simulink model "NeuronalNetwork"  (R2019b)
(part 11 of 11)

  dotprod426/1 -> Mux/426
  "IW{2,1}(427,:)'"/1 -> dotprod427/1
  dotprod427/1 -> Mux/427
  "IW{2,1}(428,:)'"/1 -> dotprod428/1
  dotprod428/1 -> Mux/428
  "IW{2,1}(429,:)'"/1 -> dotprod429/1
  dotprod429/1 -> Mux/429
  "IW{2,1}(430,:)'"/1 -> dotprod430/1
  dotprod430/1 -> Mux/430
  "IW{2,1}(431,:)'"/1 -> dotprod431/1
  dotprod431/1 -> Mux/431
  "IW{2,1}(432,:)'"/1 -> dotprod432/1
  dotprod432/1 -> Mux/432
  "IW{2,1}(433,:)'"/1 -> dotprod433/1
  dotprod433/1 -> Mux/433
  "IW{2,1}(434,:)'"/1 -> dotprod434/1
  dotprod434/1 -> Mux/434
  "IW{2,1}(435,:)'"/1 -> dotprod435/1
  dotprod435/1 -> Mux/435
  "IW{2,1}(436,:)'"/1 -> dotprod436/1
  dotprod436/1 -> Mux/436
  "IW{2,1}(437,:)'"/1 -> dotprod437/1
  dotprod437/1 -> Mux/437
  "IW{2,1}(438,:)'"/1 -> dotprod438/1
  dotprod438/1 -> Mux/438
  "IW{2,1}(439,:)'"/1 -> dotprod439/1
  dotprod439/1 -> Mux/439
  "IW{2,1}(440,:)'"/1 -> dotprod440/1
  dotprod440/1 -> Mux/440
  "IW{2,1}(441,:)'"/1 -> dotprod441/1
  dotprod441/1 -> Mux/441
  "IW{2,1}(442,:)'"/1 -> dotprod442/1
  dotprod442/1 -> Mux/442
  "IW{2,1}(443,:)'"/1 -> dotprod443/1
  dotprod443/1 -> Mux/443
  "IW{2,1}(444,:)'"/1 -> dotprod444/1
  dotprod444/1 -> Mux/444
  "IW{2,1}(445,:)'"/1 -> dotprod445/1
  dotprod445/1 -> Mux/445
  "IW{2,1}(446,:)'"/1 -> dotprod446/1
  dotprod446/1 -> Mux/446
  "IW{2,1}(447,:)'"/1 -> dotprod447/1
  dotprod447/1 -> Mux/447
  "IW{2,1}(448,:)'"/1 -> dotprod448/1
  dotprod448/1 -> Mux/448
  "IW{2,1}(449,:)'"/1 -> dotprod449/1
  dotprod449/1 -> Mux/449
  "IW{2,1}(450,:)'"/1 -> dotprod450/1
  dotprod450/1 -> Mux/450
  "IW{2,1}(451,:)'"/1 -> dotprod451/1
  dotprod451/1 -> Mux/451
  "IW{2,1}(452,:)'"/1 -> dotprod452/1
  dotprod452/1 -> Mux/452
  "IW{2,1}(453,:)'"/1 -> dotprod453/1
  dotprod453/1 -> Mux/453
  "IW{2,1}(454,:)'"/1 -> dotprod454/1
  dotprod454/1 -> Mux/454
  "IW{2,1}(455,:)'"/1 -> dotprod455/1
  dotprod455/1 -> Mux/455
  "IW{2,1}(456,:)'"/1 -> dotprod456/1
  dotprod456/1 -> Mux/456
  "IW{2,1}(457,:)'"/1 -> dotprod457/1
  dotprod457/1 -> Mux/457
  "IW{2,1}(458,:)'"/1 -> dotprod458/1
  dotprod458/1 -> Mux/458
  "IW{2,1}(459,:)'"/1 -> dotprod459/1
  dotprod459/1 -> Mux/459
  "IW{2,1}(460,:)'"/1 -> dotprod460/1
  dotprod460/1 -> Mux/460
  "IW{2,1}(461,:)'"/1 -> dotprod461/1
  dotprod461/1 -> Mux/461
  "IW{2,1}(462,:)'"/1 -> dotprod462/1
  dotprod462/1 -> Mux/462
  "IW{2,1}(463,:)'"/1 -> dotprod463/1
  dotprod463/1 -> Mux/463
  "IW{2,1}(464,:)'"/1 -> dotprod464/1
  dotprod464/1 -> Mux/464
  "IW{2,1}(465,:)'"/1 -> dotprod465/1
  dotprod465/1 -> Mux/465
  "IW{2,1}(466,:)'"/1 -> dotprod466/1
  dotprod466/1 -> Mux/466
  "IW{2,1}(467,:)'"/1 -> dotprod467/1
  dotprod467/1 -> Mux/467
  "IW{2,1}(468,:)'"/1 -> dotprod468/1
  dotprod468/1 -> Mux/468
  "IW{2,1}(469,:)'"/1 -> dotprod469/1
  dotprod469/1 -> Mux/469
  "IW{2,1}(470,:)'"/1 -> dotprod470/1
  dotprod470/1 -> Mux/470
  "IW{2,1}(471,:)'"/1 -> dotprod471/1
  dotprod471/1 -> Mux/471
  "IW{2,1}(472,:)'"/1 -> dotprod472/1
  dotprod472/1 -> Mux/472
  "IW{2,1}(473,:)'"/1 -> dotprod473/1
  dotprod473/1 -> Mux/473
  "IW{2,1}(474,:)'"/1 -> dotprod474/1
  dotprod474/1 -> Mux/474
  "IW{2,1}(475,:)'"/1 -> dotprod475/1
  dotprod475/1 -> Mux/475
  "IW{2,1}(476,:)'"/1 -> dotprod476/1
  dotprod476/1 -> Mux/476
  "IW{2,1}(477,:)'"/1 -> dotprod477/1
  dotprod477/1 -> Mux/477
  "IW{2,1}(478,:)'"/1 -> dotprod478/1
  dotprod478/1 -> Mux/478
  "IW{2,1}(479,:)'"/1 -> dotprod479/1
  dotprod479/1 -> Mux/479
  "IW{2,1}(480,:)'"/1 -> dotprod480/1
  dotprod480/1 -> Mux/480
  "IW{2,1}(481,:)'"/1 -> dotprod481/1
  dotprod481/1 -> Mux/481
  "IW{2,1}(482,:)'"/1 -> dotprod482/1
  dotprod482/1 -> Mux/482
  "IW{2,1}(483,:)'"/1 -> dotprod483/1
  dotprod483/1 -> Mux/483
  "IW{2,1}(484,:)'"/1 -> dotprod484/1
  dotprod484/1 -> Mux/484
  "IW{2,1}(485,:)'"/1 -> dotprod485/1
  dotprod485/1 -> Mux/485
  "IW{2,1}(486,:)'"/1 -> dotprod486/1
  dotprod486/1 -> Mux/486
  "IW{2,1}(487,:)'"/1 -> dotprod487/1
  dotprod487/1 -> Mux/487
  "IW{2,1}(488,:)'"/1 -> dotprod488/1
  dotprod488/1 -> Mux/488
  "IW{2,1}(489,:)'"/1 -> dotprod489/1
  dotprod489/1 -> Mux/489
  "IW{2,1}(490,:)'"/1 -> dotprod490/1
  dotprod490/1 -> Mux/490
  "IW{2,1}(491,:)'"/1 -> dotprod491/1
  dotprod491/1 -> Mux/491
  "IW{2,1}(492,:)'"/1 -> dotprod492/1
  dotprod492/1 -> Mux/492
  "IW{2,1}(493,:)'"/1 -> dotprod493/1
  dotprod493/1 -> Mux/493
  "IW{2,1}(494,:)'"/1 -> dotprod494/1
  dotprod494/1 -> Mux/494
  "IW{2,1}(495,:)'"/1 -> dotprod495/1
  dotprod495/1 -> Mux/495
  "IW{2,1}(496,:)'"/1 -> dotprod496/1
  dotprod496/1 -> Mux/496
  "IW{2,1}(497,:)'"/1 -> dotprod497/1
  dotprod497/1 -> Mux/497
  "IW{2,1}(498,:)'"/1 -> dotprod498/1
  dotprod498/1 -> Mux/498
  "IW{2,1}(499,:)'"/1 -> dotprod499/1
  dotprod499/1 -> Mux/499
  "IW{2,1}(500,:)'"/1 -> dotprod500/1
  dotprod500/1 -> Mux/500
  "IW{2,1}(501,:)'"/1 -> dotprod501/1
  dotprod501/1 -> Mux/501
  "IW{2,1}(502,:)'"/1 -> dotprod502/1
  dotprod502/1 -> Mux/502
  "IW{2,1}(503,:)'"/1 -> dotprod503/1
  dotprod503/1 -> Mux/503
  "IW{2,1}(504,:)'"/1 -> dotprod504/1
  dotprod504/1 -> Mux/504
  "IW{2,1}(505,:)'"/1 -> dotprod505/1
  dotprod505/1 -> Mux/505
  "IW{2,1}(506,:)'"/1 -> dotprod506/1
  dotprod506/1 -> Mux/506
  "IW{2,1}(507,:)'"/1 -> dotprod507/1
  dotprod507/1 -> Mux/507
  "IW{2,1}(508,:)'"/1 -> dotprod508/1
  dotprod508/1 -> Mux/508
  "IW{2,1}(509,:)'"/1 -> dotprod509/1
  dotprod509/1 -> Mux/509
  "IW{2,1}(510,:)'"/1 -> dotprod510/1
  dotprod510/1 -> Mux/510
  "IW{2,1}(511,:)'"/1 -> dotprod511/1
  dotprod511/1 -> Mux/511
  "IW{2,1}(512,:)'"/1 -> dotprod512/1
  dotprod512/1 -> Mux/512
  "IW{2,1}(513,:)'"/1 -> dotprod513/1
  dotprod513/1 -> Mux/513
  "IW{2,1}(514,:)'"/1 -> dotprod514/1
  dotprod514/1 -> Mux/514
  "IW{2,1}(515,:)'"/1 -> dotprod515/1
  dotprod515/1 -> Mux/515
  "IW{2,1}(516,:)'"/1 -> dotprod516/1
  dotprod516/1 -> Mux/516
  "IW{2,1}(517,:)'"/1 -> dotprod517/1
  dotprod517/1 -> Mux/517
  "IW{2,1}(518,:)'"/1 -> dotprod518/1
  dotprod518/1 -> Mux/518
  "IW{2,1}(519,:)'"/1 -> dotprod519/1
  dotprod519/1 -> Mux/519
  "IW{2,1}(520,:)'"/1 -> dotprod520/1
  dotprod520/1 -> Mux/520
  "IW{2,1}(521,:)'"/1 -> dotprod521/1
  dotprod521/1 -> Mux/521
  "IW{2,1}(522,:)'"/1 -> dotprod522/1
  dotprod522/1 -> Mux/522
  "IW{2,1}(523,:)'"/1 -> dotprod523/1
  dotprod523/1 -> Mux/523
  "IW{2,1}(524,:)'"/1 -> dotprod524/1
  dotprod524/1 -> Mux/524
  "IW{2,1}(525,:)'"/1 -> dotprod525/1
  dotprod525/1 -> Mux/525
  "IW{2,1}(526,:)'"/1 -> dotprod526/1
  dotprod526/1 -> Mux/526
  "IW{2,1}(527,:)'"/1 -> dotprod527/1
  dotprod527/1 -> Mux/527
  "IW{2,1}(528,:)'"/1 -> dotprod528/1
  dotprod528/1 -> Mux/528
  "IW{2,1}(529,:)'"/1 -> dotprod529/1
  dotprod529/1 -> Mux/529
  "IW{2,1}(530,:)'"/1 -> dotprod530/1
  dotprod530/1 -> Mux/530
  "IW{2,1}(531,:)'"/1 -> dotprod531/1
  dotprod531/1 -> Mux/531
  "IW{2,1}(532,:)'"/1 -> dotprod532/1
  dotprod532/1 -> Mux/532
  "IW{2,1}(533,:)'"/1 -> dotprod533/1
  dotprod533/1 -> Mux/533
  "IW{2,1}(534,:)'"/1 -> dotprod534/1
  dotprod534/1 -> Mux/534
  "IW{2,1}(535,:)'"/1 -> dotprod535/1
  dotprod535/1 -> Mux/535
  "IW{2,1}(536,:)'"/1 -> dotprod536/1
  dotprod536/1 -> Mux/536
  "IW{2,1}(537,:)'"/1 -> dotprod537/1
  dotprod537/1 -> Mux/537
  "IW{2,1}(538,:)'"/1 -> dotprod538/1
  dotprod538/1 -> Mux/538
  "IW{2,1}(539,:)'"/1 -> dotprod539/1
  dotprod539/1 -> Mux/539
  "IW{2,1}(540,:)'"/1 -> dotprod540/1
  dotprod540/1 -> Mux/540
  "IW{2,1}(541,:)'"/1 -> dotprod541/1
  dotprod541/1 -> Mux/541
  "IW{2,1}(542,:)'"/1 -> dotprod542/1
  dotprod542/1 -> Mux/542
  "IW{2,1}(543,:)'"/1 -> dotprod543/1
  dotprod543/1 -> Mux/543
  "IW{2,1}(544,:)'"/1 -> dotprod544/1
  dotprod544/1 -> Mux/544
  "IW{2,1}(545,:)'"/1 -> dotprod545/1
  dotprod545/1 -> Mux/545
  "IW{2,1}(546,:)'"/1 -> dotprod546/1
  dotprod546/1 -> Mux/546
  "IW{2,1}(547,:)'"/1 -> dotprod547/1
  dotprod547/1 -> Mux/547
  "IW{2,1}(548,:)'"/1 -> dotprod548/1
  dotprod548/1 -> Mux/548
  "IW{2,1}(549,:)'"/1 -> dotprod549/1
  dotprod549/1 -> Mux/549
  "IW{2,1}(550,:)'"/1 -> dotprod550/1
  dotprod550/1 -> Mux/550
  "IW{2,1}(551,:)'"/1 -> dotprod551/1
  dotprod551/1 -> Mux/551
  "IW{2,1}(552,:)'"/1 -> dotprod552/1
  dotprod552/1 -> Mux/552
  "IW{2,1}(553,:)'"/1 -> dotprod553/1
  dotprod553/1 -> Mux/553
  "IW{2,1}(554,:)'"/1 -> dotprod554/1
  dotprod554/1 -> Mux/554
  "IW{2,1}(555,:)'"/1 -> dotprod555/1
  dotprod555/1 -> Mux/555
  "IW{2,1}(556,:)'"/1 -> dotprod556/1
  dotprod556/1 -> Mux/556
  "IW{2,1}(557,:)'"/1 -> dotprod557/1
  dotprod557/1 -> Mux/557
  "IW{2,1}(558,:)'"/1 -> dotprod558/1
  dotprod558/1 -> Mux/558
  "IW{2,1}(559,:)'"/1 -> dotprod559/1
  dotprod559/1 -> Mux/559
  "IW{2,1}(560,:)'"/1 -> dotprod560/1
  dotprod560/1 -> Mux/560
  "IW{2,1}(561,:)'"/1 -> dotprod561/1
  dotprod561/1 -> Mux/561
  "IW{2,1}(562,:)'"/1 -> dotprod562/1
  dotprod562/1 -> Mux/562
  "IW{2,1}(563,:)'"/1 -> dotprod563/1
  dotprod563/1 -> Mux/563
  "IW{2,1}(564,:)'"/1 -> dotprod564/1
  dotprod564/1 -> Mux/564
  "IW{2,1}(565,:)'"/1 -> dotprod565/1
  dotprod565/1 -> Mux/565
  "IW{2,1}(566,:)'"/1 -> dotprod566/1
  dotprod566/1 -> Mux/566
  "IW{2,1}(567,:)'"/1 -> dotprod567/1
  dotprod567/1 -> Mux/567
  "IW{2,1}(568,:)'"/1 -> dotprod568/1
  dotprod568/1 -> Mux/568
  "IW{2,1}(569,:)'"/1 -> dotprod569/1
  dotprod569/1 -> Mux/569
  "IW{2,1}(570,:)'"/1 -> dotprod570/1
  dotprod570/1 -> Mux/570
  "IW{2,1}(571,:)'"/1 -> dotprod571/1
  dotprod571/1 -> Mux/571
  "IW{2,1}(572,:)'"/1 -> dotprod572/1
  dotprod572/1 -> Mux/572
  "IW{2,1}(573,:)'"/1 -> dotprod573/1
  dotprod573/1 -> Mux/573
  "IW{2,1}(574,:)'"/1 -> dotprod574/1
  dotprod574/1 -> Mux/574
  "IW{2,1}(575,:)'"/1 -> dotprod575/1
  dotprod575/1 -> Mux/575
  "IW{2,1}(576,:)'"/1 -> dotprod576/1
  dotprod576/1 -> Mux/576
  "IW{2,1}(577,:)'"/1 -> dotprod577/1
  dotprod577/1 -> Mux/577
  "IW{2,1}(578,:)'"/1 -> dotprod578/1
  dotprod578/1 -> Mux/578
  "IW{2,1}(579,:)'"/1 -> dotprod579/1
  dotprod579/1 -> Mux/579
  "IW{2,1}(580,:)'"/1 -> dotprod580/1
  dotprod580/1 -> Mux/580
  "IW{2,1}(581,:)'"/1 -> dotprod581/1
  dotprod581/1 -> Mux/581
  "IW{2,1}(582,:)'"/1 -> dotprod582/1
  dotprod582/1 -> Mux/582
  "IW{2,1}(583,:)'"/1 -> dotprod583/1
  dotprod583/1 -> Mux/583
  "IW{2,1}(584,:)'"/1 -> dotprod584/1
  dotprod584/1 -> Mux/584
  "IW{2,1}(585,:)'"/1 -> dotprod585/1
  dotprod585/1 -> Mux/585
  "IW{2,1}(586,:)'"/1 -> dotprod586/1
  dotprod586/1 -> Mux/586
  "IW{2,1}(587,:)'"/1 -> dotprod587/1
  dotprod587/1 -> Mux/587
  "IW{2,1}(588,:)'"/1 -> dotprod588/1
  dotprod588/1 -> Mux/588
  "IW{2,1}(589,:)'"/1 -> dotprod589/1
  dotprod589/1 -> Mux/589
  "IW{2,1}(590,:)'"/1 -> dotprod590/1
  dotprod590/1 -> Mux/590
  "IW{2,1}(591,:)'"/1 -> dotprod591/1
  dotprod591/1 -> Mux/591
  "IW{2,1}(592,:)'"/1 -> dotprod592/1
  dotprod592/1 -> Mux/592
  "IW{2,1}(593,:)'"/1 -> dotprod593/1
  dotprod593/1 -> Mux/593
  "IW{2,1}(594,:)'"/1 -> dotprod594/1
  dotprod594/1 -> Mux/594
  "IW{2,1}(595,:)'"/1 -> dotprod595/1
  dotprod595/1 -> Mux/595
  "IW{2,1}(596,:)'"/1 -> dotprod596/1
  dotprod596/1 -> Mux/596
  "IW{2,1}(597,:)'"/1 -> dotprod597/1
  dotprod597/1 -> Mux/597
  "IW{2,1}(598,:)'"/1 -> dotprod598/1
  dotprod598/1 -> Mux/598
  "IW{2,1}(599,:)'"/1 -> dotprod599/1
  dotprod599/1 -> Mux/599
  "IW{2,1}(600,:)'"/1 -> dotprod600/1
  dotprod600/1 -> Mux/600
  "IW{2,1}(601,:)'"/1 -> dotprod601/1
  dotprod601/1 -> Mux/601
  "IW{2,1}(602,:)'"/1 -> dotprod602/1
  dotprod602/1 -> Mux/602
  "IW{2,1}(603,:)'"/1 -> dotprod603/1
  dotprod603/1 -> Mux/603
  "IW{2,1}(604,:)'"/1 -> dotprod604/1
  dotprod604/1 -> Mux/604
  "IW{2,1}(605,:)'"/1 -> dotprod605/1
  dotprod605/1 -> Mux/605
  "IW{2,1}(606,:)'"/1 -> dotprod606/1
  dotprod606/1 -> Mux/606
  "IW{2,1}(607,:)'"/1 -> dotprod607/1
  dotprod607/1 -> Mux/607
  "IW{2,1}(608,:)'"/1 -> dotprod608/1
  dotprod608/1 -> Mux/608
  "IW{2,1}(609,:)'"/1 -> dotprod609/1
  dotprod609/1 -> Mux/609
  "IW{2,1}(610,:)'"/1 -> dotprod610/1
  dotprod610/1 -> Mux/610
  "IW{2,1}(611,:)'"/1 -> dotprod611/1
  dotprod611/1 -> Mux/611
  "IW{2,1}(612,:)'"/1 -> dotprod612/1
  dotprod612/1 -> Mux/612
  "IW{2,1}(613,:)'"/1 -> dotprod613/1
  dotprod613/1 -> Mux/613
  "IW{2,1}(614,:)'"/1 -> dotprod614/1
  dotprod614/1 -> Mux/614
  "IW{2,1}(615,:)'"/1 -> dotprod615/1
  dotprod615/1 -> Mux/615
  "IW{2,1}(616,:)'"/1 -> dotprod616/1
  dotprod616/1 -> Mux/616
  "IW{2,1}(617,:)'"/1 -> dotprod617/1
  dotprod617/1 -> Mux/617
  "IW{2,1}(618,:)'"/1 -> dotprod618/1
  dotprod618/1 -> Mux/618
  "IW{2,1}(619,:)'"/1 -> dotprod619/1
  dotprod619/1 -> Mux/619
  "IW{2,1}(620,:)'"/1 -> dotprod620/1
  dotprod620/1 -> Mux/620
  "IW{2,1}(621,:)'"/1 -> dotprod621/1
  dotprod621/1 -> Mux/621
  "IW{2,1}(622,:)'"/1 -> dotprod622/1
  dotprod622/1 -> Mux/622
  "IW{2,1}(623,:)'"/1 -> dotprod623/1
  dotprod623/1 -> Mux/623
  "IW{2,1}(624,:)'"/1 -> dotprod624/1
  dotprod624/1 -> Mux/624
  "IW{2,1}(625,:)'"/1 -> dotprod625/1
  dotprod625/1 -> Mux/625
  "IW{2,1}(626,:)'"/1 -> dotprod626/1
  dotprod626/1 -> Mux/626
  "IW{2,1}(627,:)'"/1 -> dotprod627/1
  dotprod627/1 -> Mux/627
  "IW{2,1}(628,:)'"/1 -> dotprod628/1
  dotprod628/1 -> Mux/628
  "IW{2,1}(629,:)'"/1 -> dotprod629/1
  dotprod629/1 -> Mux/629
  "IW{2,1}(630,:)'"/1 -> dotprod630/1
  dotprod630/1 -> Mux/630
  "IW{2,1}(631,:)'"/1 -> dotprod631/1
  dotprod631/1 -> Mux/631
  "IW{2,1}(632,:)'"/1 -> dotprod632/1
  dotprod632/1 -> Mux/632
  "IW{2,1}(633,:)'"/1 -> dotprod633/1
  dotprod633/1 -> Mux/633
  "IW{2,1}(634,:)'"/1 -> dotprod634/1
  dotprod634/1 -> Mux/634
  "IW{2,1}(635,:)'"/1 -> dotprod635/1
  dotprod635/1 -> Mux/635
  "IW{2,1}(636,:)'"/1 -> dotprod636/1
  dotprod636/1 -> Mux/636
  "IW{2,1}(637,:)'"/1 -> dotprod637/1
  dotprod637/1 -> Mux/637
  "IW{2,1}(638,:)'"/1 -> dotprod638/1
  dotprod638/1 -> Mux/638
  "IW{2,1}(639,:)'"/1 -> dotprod639/1
  dotprod639/1 -> Mux/639
  "IW{2,1}(640,:)'"/1 -> dotprod640/1
  dotprod640/1 -> Mux/640
  "IW{2,1}(641,:)'"/1 -> dotprod641/1
  dotprod641/1 -> Mux/641
  "IW{2,1}(642,:)'"/1 -> dotprod642/1
  dotprod642/1 -> Mux/642
  "IW{2,1}(643,:)'"/1 -> dotprod643/1
  dotprod643/1 -> Mux/643
  "IW{2,1}(644,:)'"/1 -> dotprod644/1
  dotprod644/1 -> Mux/644
  "IW{2,1}(645,:)'"/1 -> dotprod645/1
  dotprod645/1 -> Mux/645
  "IW{2,1}(646,:)'"/1 -> dotprod646/1
  dotprod646/1 -> Mux/646
  "IW{2,1}(647,:)'"/1 -> dotprod647/1
  dotprod647/1 -> Mux/647
  "IW{2,1}(648,:)'"/1 -> dotprod648/1
  dotprod648/1 -> Mux/648
  "IW{2,1}(649,:)'"/1 -> dotprod649/1
  dotprod649/1 -> Mux/649
  "IW{2,1}(650,:)'"/1 -> dotprod650/1
  dotprod650/1 -> Mux/650
  "IW{2,1}(651,:)'"/1 -> dotprod651/1
  dotprod651/1 -> Mux/651
  "IW{2,1}(652,:)'"/1 -> dotprod652/1
  dotprod652/1 -> Mux/652
  "IW{2,1}(653,:)'"/1 -> dotprod653/1
  dotprod653/1 -> Mux/653
  "IW{2,1}(654,:)'"/1 -> dotprod654/1
  dotprod654/1 -> Mux/654
  "IW{2,1}(655,:)'"/1 -> dotprod655/1
  dotprod655/1 -> Mux/655
  "IW{2,1}(656,:)'"/1 -> dotprod656/1
  dotprod656/1 -> Mux/656
  "IW{2,1}(657,:)'"/1 -> dotprod657/1
  dotprod657/1 -> Mux/657
  "IW{2,1}(658,:)'"/1 -> dotprod658/1
  dotprod658/1 -> Mux/658
  "IW{2,1}(659,:)'"/1 -> dotprod659/1
  dotprod659/1 -> Mux/659
  "IW{2,1}(660,:)'"/1 -> dotprod660/1
  dotprod660/1 -> Mux/660
  "IW{2,1}(661,:)'"/1 -> dotprod661/1
  dotprod661/1 -> Mux/661
  "IW{2,1}(662,:)'"/1 -> dotprod662/1
  dotprod662/1 -> Mux/662
  "IW{2,1}(663,:)'"/1 -> dotprod663/1
  dotprod663/1 -> Mux/663
  "IW{2,1}(664,:)'"/1 -> dotprod664/1
  dotprod664/1 -> Mux/664
  "IW{2,1}(665,:)'"/1 -> dotprod665/1
  dotprod665/1 -> Mux/665
  "IW{2,1}(666,:)'"/1 -> dotprod666/1
  dotprod666/1 -> Mux/666
  "IW{2,1}(667,:)'"/1 -> dotprod667/1
  dotprod667/1 -> Mux/667
  "IW{2,1}(668,:)'"/1 -> dotprod668/1
  dotprod668/1 -> Mux/668
  "IW{2,1}(669,:)'"/1 -> dotprod669/1
  dotprod669/1 -> Mux/669
  "IW{2,1}(670,:)'"/1 -> dotprod670/1
  dotprod670/1 -> Mux/670
  "IW{2,1}(671,:)'"/1 -> dotprod671/1
  dotprod671/1 -> Mux/671
  "IW{2,1}(672,:)'"/1 -> dotprod672/1
  dotprod672/1 -> Mux/672
  "IW{2,1}(673,:)'"/1 -> dotprod673/1
  dotprod673/1 -> Mux/673
  "IW{2,1}(674,:)'"/1 -> dotprod674/1
  dotprod674/1 -> Mux/674
  "IW{2,1}(675,:)'"/1 -> dotprod675/1
  dotprod675/1 -> Mux/675
  "IW{2,1}(676,:)'"/1 -> dotprod676/1
  dotprod676/1 -> Mux/676
  "IW{2,1}(677,:)'"/1 -> dotprod677/1
  dotprod677/1 -> Mux/677
  "IW{2,1}(678,:)'"/1 -> dotprod678/1
  dotprod678/1 -> Mux/678
  "IW{2,1}(679,:)'"/1 -> dotprod679/1
  dotprod679/1 -> Mux/679
  "IW{2,1}(680,:)'"/1 -> dotprod680/1
  dotprod680/1 -> Mux/680
  "IW{2,1}(681,:)'"/1 -> dotprod681/1
  dotprod681/1 -> Mux/681
  "IW{2,1}(682,:)'"/1 -> dotprod682/1
  dotprod682/1 -> Mux/682
  "IW{2,1}(683,:)'"/1 -> dotprod683/1
  dotprod683/1 -> Mux/683
  "IW{2,1}(684,:)'"/1 -> dotprod684/1
  dotprod684/1 -> Mux/684
  "IW{2,1}(685,:)'"/1 -> dotprod685/1
  dotprod685/1 -> Mux/685
  "IW{2,1}(686,:)'"/1 -> dotprod686/1
  dotprod686/1 -> Mux/686
  "IW{2,1}(687,:)'"/1 -> dotprod687/1
  dotprod687/1 -> Mux/687
  "IW{2,1}(688,:)'"/1 -> dotprod688/1
  dotprod688/1 -> Mux/688
  "IW{2,1}(689,:)'"/1 -> dotprod689/1
  dotprod689/1 -> Mux/689
  "IW{2,1}(690,:)'"/1 -> dotprod690/1
  dotprod690/1 -> Mux/690
  "IW{2,1}(691,:)'"/1 -> dotprod691/1
  dotprod691/1 -> Mux/691
  "IW{2,1}(692,:)'"/1 -> dotprod692/1
  dotprod692/1 -> Mux/692
  "IW{2,1}(693,:)'"/1 -> dotprod693/1
  dotprod693/1 -> Mux/693
  "IW{2,1}(694,:)'"/1 -> dotprod694/1
  dotprod694/1 -> Mux/694
  "IW{2,1}(695,:)'"/1 -> dotprod695/1
  dotprod695/1 -> Mux/695
  "IW{2,1}(696,:)'"/1 -> dotprod696/1
  dotprod696/1 -> Mux/696
  "IW{2,1}(697,:)'"/1 -> dotprod697/1
  dotprod697/1 -> Mux/697
  "IW{2,1}(698,:)'"/1 -> dotprod698/1
  dotprod698/1 -> Mux/698
  "IW{2,1}(699,:)'"/1 -> dotprod699/1
  dotprod699/1 -> Mux/699
  "IW{2,1}(700,:)'"/1 -> dotprod700/1
  dotprod700/1 -> Mux/700
  "IW{2,1}(701,:)'"/1 -> dotprod701/1
  dotprod701/1 -> Mux/701
  "IW{2,1}(702,:)'"/1 -> dotprod702/1
  dotprod702/1 -> Mux/702
  "IW{2,1}(703,:)'"/1 -> dotprod703/1
  dotprod703/1 -> Mux/703
  "IW{2,1}(704,:)'"/1 -> dotprod704/1
  dotprod704/1 -> Mux/704
  "IW{2,1}(705,:)'"/1 -> dotprod705/1
  dotprod705/1 -> Mux/705
  "IW{2,1}(706,:)'"/1 -> dotprod706/1
  dotprod706/1 -> Mux/706
  "IW{2,1}(707,:)'"/1 -> dotprod707/1
  dotprod707/1 -> Mux/707
  "IW{2,1}(708,:)'"/1 -> dotprod708/1
  dotprod708/1 -> Mux/708
  "IW{2,1}(709,:)'"/1 -> dotprod709/1
  dotprod709/1 -> Mux/709
  "IW{2,1}(710,:)'"/1 -> dotprod710/1
  dotprod710/1 -> Mux/710
  "IW{2,1}(711,:)'"/1 -> dotprod711/1
  dotprod711/1 -> Mux/711
  "IW{2,1}(712,:)'"/1 -> dotprod712/1
  dotprod712/1 -> Mux/712
  "IW{2,1}(713,:)'"/1 -> dotprod713/1
  dotprod713/1 -> Mux/713
  "IW{2,1}(714,:)'"/1 -> dotprod714/1
  dotprod714/1 -> Mux/714
  "IW{2,1}(715,:)'"/1 -> dotprod715/1
  dotprod715/1 -> Mux/715
  "IW{2,1}(716,:)'"/1 -> dotprod716/1
  dotprod716/1 -> Mux/716
  "IW{2,1}(717,:)'"/1 -> dotprod717/1
  dotprod717/1 -> Mux/717
  "IW{2,1}(718,:)'"/1 -> dotprod718/1
  dotprod718/1 -> Mux/718
  "IW{2,1}(719,:)'"/1 -> dotprod719/1
  dotprod719/1 -> Mux/719
  "IW{2,1}(720,:)'"/1 -> dotprod720/1
  dotprod720/1 -> Mux/720
  "IW{2,1}(721,:)'"/1 -> dotprod721/1
  dotprod721/1 -> Mux/721
  "IW{2,1}(722,:)'"/1 -> dotprod722/1
  dotprod722/1 -> Mux/722
  "IW{2,1}(723,:)'"/1 -> dotprod723/1
  dotprod723/1 -> Mux/723
  "IW{2,1}(724,:)'"/1 -> dotprod724/1
  dotprod724/1 -> Mux/724
  "IW{2,1}(725,:)'"/1 -> dotprod725/1
  dotprod725/1 -> Mux/725
  "IW{2,1}(726,:)'"/1 -> dotprod726/1
  dotprod726/1 -> Mux/726
  "IW{2,1}(727,:)'"/1 -> dotprod727/1
  dotprod727/1 -> Mux/727
  "IW{2,1}(728,:)'"/1 -> dotprod728/1
  dotprod728/1 -> Mux/728
  "IW{2,1}(729,:)'"/1 -> dotprod729/1
  dotprod729/1 -> Mux/729
  "IW{2,1}(730,:)'"/1 -> dotprod730/1
  dotprod730/1 -> Mux/730
  "IW{2,1}(731,:)'"/1 -> dotprod731/1
  dotprod731/1 -> Mux/731
  "IW{2,1}(732,:)'"/1 -> dotprod732/1
  dotprod732/1 -> Mux/732
  "IW{2,1}(733,:)'"/1 -> dotprod733/1
  dotprod733/1 -> Mux/733
  "IW{2,1}(734,:)'"/1 -> dotprod734/1
  dotprod734/1 -> Mux/734
  "IW{2,1}(735,:)'"/1 -> dotprod735/1
  dotprod735/1 -> Mux/735
  "IW{2,1}(736,:)'"/1 -> dotprod736/1
  dotprod736/1 -> Mux/736
  "IW{2,1}(737,:)'"/1 -> dotprod737/1
  dotprod737/1 -> Mux/737
  "IW{2,1}(738,:)'"/1 -> dotprod738/1
  dotprod738/1 -> Mux/738
  "IW{2,1}(739,:)'"/1 -> dotprod739/1
  dotprod739/1 -> Mux/739
  "IW{2,1}(740,:)'"/1 -> dotprod740/1
  dotprod740/1 -> Mux/740
  "IW{2,1}(741,:)'"/1 -> dotprod741/1
  dotprod741/1 -> Mux/741
  "IW{2,1}(742,:)'"/1 -> dotprod742/1
  dotprod742/1 -> Mux/742
  "IW{2,1}(743,:)'"/1 -> dotprod743/1
  dotprod743/1 -> Mux/743
  "IW{2,1}(744,:)'"/1 -> dotprod744/1
  dotprod744/1 -> Mux/744
  "IW{2,1}(745,:)'"/1 -> dotprod745/1
  dotprod745/1 -> Mux/745
  "IW{2,1}(746,:)'"/1 -> dotprod746/1
  dotprod746/1 -> Mux/746
  "IW{2,1}(747,:)'"/1 -> dotprod747/1
  dotprod747/1 -> Mux/747
  "IW{2,1}(748,:)'"/1 -> dotprod748/1
  dotprod748/1 -> Mux/748
  "IW{2,1}(749,:)'"/1 -> dotprod749/1
  dotprod749/1 -> Mux/749
  "IW{2,1}(750,:)'"/1 -> dotprod750/1
  dotprod750/1 -> Mux/750
  "IW{2,1}(751,:)'"/1 -> dotprod751/1
  dotprod751/1 -> Mux/751
  "IW{2,1}(752,:)'"/1 -> dotprod752/1
  dotprod752/1 -> Mux/752
  "IW{2,1}(753,:)'"/1 -> dotprod753/1
  dotprod753/1 -> Mux/753
  "IW{2,1}(754,:)'"/1 -> dotprod754/1
  dotprod754/1 -> Mux/754
  "IW{2,1}(755,:)'"/1 -> dotprod755/1
  dotprod755/1 -> Mux/755
  "IW{2,1}(756,:)'"/1 -> dotprod756/1
  dotprod756/1 -> Mux/756
  "IW{2,1}(757,:)'"/1 -> dotprod757/1
  dotprod757/1 -> Mux/757
  "IW{2,1}(758,:)'"/1 -> dotprod758/1
  dotprod758/1 -> Mux/758
  "IW{2,1}(759,:)'"/1 -> dotprod759/1
  dotprod759/1 -> Mux/759
  "IW{2,1}(760,:)'"/1 -> dotprod760/1
  dotprod760/1 -> Mux/760
  "IW{2,1}(761,:)'"/1 -> dotprod761/1
  dotprod761/1 -> Mux/761
  "IW{2,1}(762,:)'"/1 -> dotprod762/1
  dotprod762/1 -> Mux/762
  "IW{2,1}(763,:)'"/1 -> dotprod763/1
  dotprod763/1 -> Mux/763
  "IW{2,1}(764,:)'"/1 -> dotprod764/1
  dotprod764/1 -> Mux/764
  "IW{2,1}(765,:)'"/1 -> dotprod765/1
  dotprod765/1 -> Mux/765
  "IW{2,1}(766,:)'"/1 -> dotprod766/1
  dotprod766/1 -> Mux/766
  "IW{2,1}(767,:)'"/1 -> dotprod767/1
  dotprod767/1 -> Mux/767
  "IW{2,1}(768,:)'"/1 -> dotprod768/1
  dotprod768/1 -> Mux/768
  "IW{2,1}(769,:)'"/1 -> dotprod769/1
  dotprod769/1 -> Mux/769
  "IW{2,1}(770,:)'"/1 -> dotprod770/1
  dotprod770/1 -> Mux/770
  "IW{2,1}(771,:)'"/1 -> dotprod771/1
  dotprod771/1 -> Mux/771
  "IW{2,1}(772,:)'"/1 -> dotprod772/1
  dotprod772/1 -> Mux/772
  "IW{2,1}(773,:)'"/1 -> dotprod773/1
  dotprod773/1 -> Mux/773
  "IW{2,1}(774,:)'"/1 -> dotprod774/1
  dotprod774/1 -> Mux/774
  "IW{2,1}(775,:)'"/1 -> dotprod775/1
  dotprod775/1 -> Mux/775
  "IW{2,1}(776,:)'"/1 -> dotprod776/1
  dotprod776/1 -> Mux/776
  "IW{2,1}(777,:)'"/1 -> dotprod777/1
  dotprod777/1 -> Mux/777
  "IW{2,1}(778,:)'"/1 -> dotprod778/1
  dotprod778/1 -> Mux/778
  "IW{2,1}(779,:)'"/1 -> dotprod779/1
  dotprod779/1 -> Mux/779
  "IW{2,1}(780,:)'"/1 -> dotprod780/1
  dotprod780/1 -> Mux/780
  "IW{2,1}(781,:)'"/1 -> dotprod781/1
  dotprod781/1 -> Mux/781
  "IW{2,1}(782,:)'"/1 -> dotprod782/1
  dotprod782/1 -> Mux/782
  "IW{2,1}(783,:)'"/1 -> dotprod783/1
  dotprod783/1 -> Mux/783
  "IW{2,1}(784,:)'"/1 -> dotprod784/1
  dotprod784/1 -> Mux/784
  "IW{2,1}(785,:)'"/1 -> dotprod785/1
  dotprod785/1 -> Mux/785
  "IW{2,1}(786,:)'"/1 -> dotprod786/1
  dotprod786/1 -> Mux/786
  "IW{2,1}(787,:)'"/1 -> dotprod787/1
  dotprod787/1 -> Mux/787
  "IW{2,1}(788,:)'"/1 -> dotprod788/1
  dotprod788/1 -> Mux/788
  "IW{2,1}(789,:)'"/1 -> dotprod789/1
  dotprod789/1 -> Mux/789
  "IW{2,1}(790,:)'"/1 -> dotprod790/1
  dotprod790/1 -> Mux/790
  "IW{2,1}(791,:)'"/1 -> dotprod791/1
  dotprod791/1 -> Mux/791
  "IW{2,1}(792,:)'"/1 -> dotprod792/1
  dotprod792/1 -> Mux/792
  "IW{2,1}(793,:)'"/1 -> dotprod793/1
  dotprod793/1 -> Mux/793
  "IW{2,1}(794,:)'"/1 -> dotprod794/1
  dotprod794/1 -> Mux/794
  "IW{2,1}(795,:)'"/1 -> dotprod795/1
  dotprod795/1 -> Mux/795
  "IW{2,1}(796,:)'"/1 -> dotprod796/1
  dotprod796/1 -> Mux/796
  "IW{2,1}(797,:)'"/1 -> dotprod797/1
  dotprod797/1 -> Mux/797
  "IW{2,1}(798,:)'"/1 -> dotprod798/1
  dotprod798/1 -> Mux/798
  "IW{2,1}(799,:)'"/1 -> dotprod799/1
  dotprod799/1 -> Mux/799
  "IW{2,1}(800,:)'"/1 -> dotprod800/1
  dotprod800/1 -> Mux/800
  "IW{2,1}(801,:)'"/1 -> dotprod801/1
  dotprod801/1 -> Mux/801
  "IW{2,1}(802,:)'"/1 -> dotprod802/1
  dotprod802/1 -> Mux/802
  "IW{2,1}(803,:)'"/1 -> dotprod803/1
  dotprod803/1 -> Mux/803
  "IW{2,1}(804,:)'"/1 -> dotprod804/1
  dotprod804/1 -> Mux/804
  "IW{2,1}(805,:)'"/1 -> dotprod805/1
  dotprod805/1 -> Mux/805
  "IW{2,1}(806,:)'"/1 -> dotprod806/1
  dotprod806/1 -> Mux/806
  "IW{2,1}(807,:)'"/1 -> dotprod807/1
  dotprod807/1 -> Mux/807
  "IW{2,1}(808,:)'"/1 -> dotprod808/1
  dotprod808/1 -> Mux/808
  "IW{2,1}(809,:)'"/1 -> dotprod809/1
  dotprod809/1 -> Mux/809
  "IW{2,1}(810,:)'"/1 -> dotprod810/1
  dotprod810/1 -> Mux/810
  "IW{2,1}(811,:)'"/1 -> dotprod811/1
  dotprod811/1 -> Mux/811
  "IW{2,1}(812,:)'"/1 -> dotprod812/1
  dotprod812/1 -> Mux/812
  "IW{2,1}(813,:)'"/1 -> dotprod813/1
  dotprod813/1 -> Mux/813
  "IW{2,1}(814,:)'"/1 -> dotprod814/1
  dotprod814/1 -> Mux/814
  "IW{2,1}(815,:)'"/1 -> dotprod815/1
  dotprod815/1 -> Mux/815
  "IW{2,1}(816,:)'"/1 -> dotprod816/1
  dotprod816/1 -> Mux/816
  "IW{2,1}(817,:)'"/1 -> dotprod817/1
  dotprod817/1 -> Mux/817
  "IW{2,1}(818,:)'"/1 -> dotprod818/1
  dotprod818/1 -> Mux/818
  "IW{2,1}(819,:)'"/1 -> dotprod819/1
  dotprod819/1 -> Mux/819
  "IW{2,1}(820,:)'"/1 -> dotprod820/1
  dotprod820/1 -> Mux/820
  "IW{2,1}(821,:)'"/1 -> dotprod821/1
  dotprod821/1 -> Mux/821
  "IW{2,1}(822,:)'"/1 -> dotprod822/1
  dotprod822/1 -> Mux/822
  "IW{2,1}(823,:)'"/1 -> dotprod823/1
  dotprod823/1 -> Mux/823
  "IW{2,1}(824,:)'"/1 -> dotprod824/1
  dotprod824/1 -> Mux/824
  "IW{2,1}(825,:)'"/1 -> dotprod825/1
  dotprod825/1 -> Mux/825
  "IW{2,1}(826,:)'"/1 -> dotprod826/1
  dotprod826/1 -> Mux/826
  "IW{2,1}(827,:)'"/1 -> dotprod827/1
  dotprod827/1 -> Mux/827
  "IW{2,1}(828,:)'"/1 -> dotprod828/1
  dotprod828/1 -> Mux/828
  "IW{2,1}(829,:)'"/1 -> dotprod829/1
  dotprod829/1 -> Mux/829
  "IW{2,1}(830,:)'"/1 -> dotprod830/1
  dotprod830/1 -> Mux/830
  "IW{2,1}(831,:)'"/1 -> dotprod831/1
  dotprod831/1 -> Mux/831
  "IW{2,1}(832,:)'"/1 -> dotprod832/1
  dotprod832/1 -> Mux/832
  "IW{2,1}(833,:)'"/1 -> dotprod833/1
  dotprod833/1 -> Mux/833
  "IW{2,1}(834,:)'"/1 -> dotprod834/1
  dotprod834/1 -> Mux/834
  "IW{2,1}(835,:)'"/1 -> dotprod835/1
  dotprod835/1 -> Mux/835
  "IW{2,1}(836,:)'"/1 -> dotprod836/1
  dotprod836/1 -> Mux/836
  "IW{2,1}(837,:)'"/1 -> dotprod837/1
  dotprod837/1 -> Mux/837
  "IW{2,1}(838,:)'"/1 -> dotprod838/1
  dotprod838/1 -> Mux/838
  "IW{2,1}(839,:)'"/1 -> dotprod839/1
  dotprod839/1 -> Mux/839
  "IW{2,1}(840,:)'"/1 -> dotprod840/1
  dotprod840/1 -> Mux/840
  "IW{2,1}(841,:)'"/1 -> dotprod841/1
  dotprod841/1 -> Mux/841
  "IW{2,1}(842,:)'"/1 -> dotprod842/1
  dotprod842/1 -> Mux/842
  "IW{2,1}(843,:)'"/1 -> dotprod843/1
  dotprod843/1 -> Mux/843
  "IW{2,1}(844,:)'"/1 -> dotprod844/1
  dotprod844/1 -> Mux/844
  "IW{2,1}(845,:)'"/1 -> dotprod845/1
  dotprod845/1 -> Mux/845
  "IW{2,1}(846,:)'"/1 -> dotprod846/1
  dotprod846/1 -> Mux/846
  "IW{2,1}(847,:)'"/1 -> dotprod847/1
  dotprod847/1 -> Mux/847
  "IW{2,1}(848,:)'"/1 -> dotprod848/1
  dotprod848/1 -> Mux/848
  "IW{2,1}(849,:)'"/1 -> dotprod849/1
  dotprod849/1 -> Mux/849
  "IW{2,1}(850,:)'"/1 -> dotprod850/1
  dotprod850/1 -> Mux/850
  "IW{2,1}(851,:)'"/1 -> dotprod851/1
  dotprod851/1 -> Mux/851
  "IW{2,1}(852,:)'"/1 -> dotprod852/1
  dotprod852/1 -> Mux/852
  "IW{2,1}(853,:)'"/1 -> dotprod853/1
  dotprod853/1 -> Mux/853
  "IW{2,1}(854,:)'"/1 -> dotprod854/1
  dotprod854/1 -> Mux/854
  "IW{2,1}(855,:)'"/1 -> dotprod855/1
  dotprod855/1 -> Mux/855
  "IW{2,1}(856,:)'"/1 -> dotprod856/1
  dotprod856/1 -> Mux/856
  "IW{2,1}(857,:)'"/1 -> dotprod857/1
  dotprod857/1 -> Mux/857
  "IW{2,1}(858,:)'"/1 -> dotprod858/1
  dotprod858/1 -> Mux/858
  "IW{2,1}(859,:)'"/1 -> dotprod859/1
  dotprod859/1 -> Mux/859
  "IW{2,1}(860,:)'"/1 -> dotprod860/1
  dotprod860/1 -> Mux/860
  "IW{2,1}(861,:)'"/1 -> dotprod861/1
  dotprod861/1 -> Mux/861
  "IW{2,1}(862,:)'"/1 -> dotprod862/1
  dotprod862/1 -> Mux/862
  "IW{2,1}(863,:)'"/1 -> dotprod863/1
  dotprod863/1 -> Mux/863
  "IW{2,1}(864,:)'"/1 -> dotprod864/1
  dotprod864/1 -> Mux/864
  "IW{2,1}(865,:)'"/1 -> dotprod865/1
  dotprod865/1 -> Mux/865
  "IW{2,1}(866,:)'"/1 -> dotprod866/1
  dotprod866/1 -> Mux/866
  "IW{2,1}(867,:)'"/1 -> dotprod867/1
  dotprod867/1 -> Mux/867
  "IW{2,1}(868,:)'"/1 -> dotprod868/1
  dotprod868/1 -> Mux/868
  "IW{2,1}(869,:)'"/1 -> dotprod869/1
  dotprod869/1 -> Mux/869
  "IW{2,1}(870,:)'"/1 -> dotprod870/1
  dotprod870/1 -> Mux/870
  "IW{2,1}(871,:)'"/1 -> dotprod871/1
  dotprod871/1 -> Mux/871
  "IW{2,1}(872,:)'"/1 -> dotprod872/1
  dotprod872/1 -> Mux/872
  "IW{2,1}(873,:)'"/1 -> dotprod873/1
  dotprod873/1 -> Mux/873
  "IW{2,1}(874,:)'"/1 -> dotprod874/1
  dotprod874/1 -> Mux/874
  "IW{2,1}(875,:)'"/1 -> dotprod875/1
  dotprod875/1 -> Mux/875
  "IW{2,1}(876,:)'"/1 -> dotprod876/1
  dotprod876/1 -> Mux/876
  "IW{2,1}(877,:)'"/1 -> dotprod877/1
  dotprod877/1 -> Mux/877
  "IW{2,1}(878,:)'"/1 -> dotprod878/1
  dotprod878/1 -> Mux/878
  "IW{2,1}(879,:)'"/1 -> dotprod879/1
  dotprod879/1 -> Mux/879
  "IW{2,1}(880,:)'"/1 -> dotprod880/1
  dotprod880/1 -> Mux/880
  "IW{2,1}(881,:)'"/1 -> dotprod881/1
  dotprod881/1 -> Mux/881
  "IW{2,1}(882,:)'"/1 -> dotprod882/1
  dotprod882/1 -> Mux/882
  "IW{2,1}(883,:)'"/1 -> dotprod883/1
  dotprod883/1 -> Mux/883
  "IW{2,1}(884,:)'"/1 -> dotprod884/1
  dotprod884/1 -> Mux/884
  "IW{2,1}(885,:)'"/1 -> dotprod885/1
  dotprod885/1 -> Mux/885
  "IW{2,1}(886,:)'"/1 -> dotprod886/1
  dotprod886/1 -> Mux/886
  "IW{2,1}(887,:)'"/1 -> dotprod887/1
  dotprod887/1 -> Mux/887
  "IW{2,1}(888,:)'"/1 -> dotprod888/1
  dotprod888/1 -> Mux/888
  "IW{2,1}(889,:)'"/1 -> dotprod889/1
  dotprod889/1 -> Mux/889
  "IW{2,1}(890,:)'"/1 -> dotprod890/1
  dotprod890/1 -> Mux/890
  "IW{2,1}(891,:)'"/1 -> dotprod891/1
  dotprod891/1 -> Mux/891
  "IW{2,1}(892,:)'"/1 -> dotprod892/1
  dotprod892/1 -> Mux/892
  "IW{2,1}(893,:)'"/1 -> dotprod893/1
  dotprod893/1 -> Mux/893
  "IW{2,1}(894,:)'"/1 -> dotprod894/1
  dotprod894/1 -> Mux/894
  "IW{2,1}(895,:)'"/1 -> dotprod895/1
  dotprod895/1 -> Mux/895
  "IW{2,1}(896,:)'"/1 -> dotprod896/1
  dotprod896/1 -> Mux/896
  "IW{2,1}(897,:)'"/1 -> dotprod897/1
  dotprod897/1 -> Mux/897
  "IW{2,1}(898,:)'"/1 -> dotprod898/1
  dotprod898/1 -> Mux/898
  "IW{2,1}(899,:)'"/1 -> dotprod899/1
  dotprod899/1 -> Mux/899
  "IW{2,1}(900,:)'"/1 -> dotprod900/1
  dotprod900/1 -> Mux/900
  "IW{2,1}(901,:)'"/1 -> dotprod901/1
  dotprod901/1 -> Mux/901
  "IW{2,1}(902,:)'"/1 -> dotprod902/1
  dotprod902/1 -> Mux/902
  "IW{2,1}(903,:)'"/1 -> dotprod903/1
  dotprod903/1 -> Mux/903
  "IW{2,1}(904,:)'"/1 -> dotprod904/1
  dotprod904/1 -> Mux/904
  "IW{2,1}(905,:)'"/1 -> dotprod905/1
  dotprod905/1 -> Mux/905
  "IW{2,1}(906,:)'"/1 -> dotprod906/1
  dotprod906/1 -> Mux/906
  "IW{2,1}(907,:)'"/1 -> dotprod907/1
  dotprod907/1 -> Mux/907
  "IW{2,1}(908,:)'"/1 -> dotprod908/1
  dotprod908/1 -> Mux/908
  "IW{2,1}(909,:)'"/1 -> dotprod909/1
  dotprod909/1 -> Mux/909
  "IW{2,1}(910,:)'"/1 -> dotprod910/1
  dotprod910/1 -> Mux/910
  "IW{2,1}(911,:)'"/1 -> dotprod911/1
  dotprod911/1 -> Mux/911
  "IW{2,1}(912,:)'"/1 -> dotprod912/1
  dotprod912/1 -> Mux/912
  "IW{2,1}(913,:)'"/1 -> dotprod913/1
  dotprod913/1 -> Mux/913
  "IW{2,1}(914,:)'"/1 -> dotprod914/1
  dotprod914/1 -> Mux/914
  "IW{2,1}(915,:)'"/1 -> dotprod915/1
  dotprod915/1 -> Mux/915
  "IW{2,1}(916,:)'"/1 -> dotprod916/1
  dotprod916/1 -> Mux/916
  "IW{2,1}(917,:)'"/1 -> dotprod917/1
  dotprod917/1 -> Mux/917
  "IW{2,1}(918,:)'"/1 -> dotprod918/1
  dotprod918/1 -> Mux/918
  "IW{2,1}(919,:)'"/1 -> dotprod919/1
  dotprod919/1 -> Mux/919
  "IW{2,1}(920,:)'"/1 -> dotprod920/1
  dotprod920/1 -> Mux/920
  "IW{2,1}(921,:)'"/1 -> dotprod921/1
  dotprod921/1 -> Mux/921
  "IW{2,1}(922,:)'"/1 -> dotprod922/1
  dotprod922/1 -> Mux/922
  "IW{2,1}(923,:)'"/1 -> dotprod923/1
  dotprod923/1 -> Mux/923
  "IW{2,1}(924,:)'"/1 -> dotprod924/1
  dotprod924/1 -> Mux/924
  "IW{2,1}(925,:)'"/1 -> dotprod925/1
  dotprod925/1 -> Mux/925
  "IW{2,1}(926,:)'"/1 -> dotprod926/1
  dotprod926/1 -> Mux/926
  "IW{2,1}(927,:)'"/1 -> dotprod927/1
  dotprod927/1 -> Mux/927
  "IW{2,1}(928,:)'"/1 -> dotprod928/1
  dotprod928/1 -> Mux/928
  "IW{2,1}(929,:)'"/1 -> dotprod929/1
  dotprod929/1 -> Mux/929
  "IW{2,1}(930,:)'"/1 -> dotprod930/1
  dotprod930/1 -> Mux/930
  "IW{2,1}(931,:)'"/1 -> dotprod931/1
  dotprod931/1 -> Mux/931
  "IW{2,1}(932,:)'"/1 -> dotprod932/1
  dotprod932/1 -> Mux/932
  "IW{2,1}(933,:)'"/1 -> dotprod933/1
  dotprod933/1 -> Mux/933
  "IW{2,1}(934,:)'"/1 -> dotprod934/1
  dotprod934/1 -> Mux/934
  "IW{2,1}(935,:)'"/1 -> dotprod935/1
  dotprod935/1 -> Mux/935
  "IW{2,1}(936,:)'"/1 -> dotprod936/1
  dotprod936/1 -> Mux/936
  "IW{2,1}(937,:)'"/1 -> dotprod937/1
  dotprod937/1 -> Mux/937
  "IW{2,1}(938,:)'"/1 -> dotprod938/1
  dotprod938/1 -> Mux/938
  "IW{2,1}(939,:)'"/1 -> dotprod939/1
  dotprod939/1 -> Mux/939
  "IW{2,1}(940,:)'"/1 -> dotprod940/1
  dotprod940/1 -> Mux/940
  "IW{2,1}(941,:)'"/1 -> dotprod941/1
  dotprod941/1 -> Mux/941
  "IW{2,1}(942,:)'"/1 -> dotprod942/1
  dotprod942/1 -> Mux/942
  "IW{2,1}(943,:)'"/1 -> dotprod943/1
  dotprod943/1 -> Mux/943
  "IW{2,1}(944,:)'"/1 -> dotprod944/1
  dotprod944/1 -> Mux/944
  "IW{2,1}(945,:)'"/1 -> dotprod945/1
  dotprod945/1 -> Mux/945
  "IW{2,1}(946,:)'"/1 -> dotprod946/1
  dotprod946/1 -> Mux/946
  "IW{2,1}(947,:)'"/1 -> dotprod947/1
  dotprod947/1 -> Mux/947
  "IW{2,1}(948,:)'"/1 -> dotprod948/1
  dotprod948/1 -> Mux/948
  "IW{2,1}(949,:)'"/1 -> dotprod949/1
  dotprod949/1 -> Mux/949
  "IW{2,1}(950,:)'"/1 -> dotprod950/1
  dotprod950/1 -> Mux/950
  "IW{2,1}(951,:)'"/1 -> dotprod951/1
  dotprod951/1 -> Mux/951
  "IW{2,1}(952,:)'"/1 -> dotprod952/1
  dotprod952/1 -> Mux/952
  "IW{2,1}(953,:)'"/1 -> dotprod953/1
  dotprod953/1 -> Mux/953
  "IW{2,1}(954,:)'"/1 -> dotprod954/1
  dotprod954/1 -> Mux/954
  "IW{2,1}(955,:)'"/1 -> dotprod955/1
  dotprod955/1 -> Mux/955
  "IW{2,1}(956,:)'"/1 -> dotprod956/1
  dotprod956/1 -> Mux/956
  "IW{2,1}(957,:)'"/1 -> dotprod957/1
  dotprod957/1 -> Mux/957
  "IW{2,1}(958,:)'"/1 -> dotprod958/1
  dotprod958/1 -> Mux/958
  "IW{2,1}(959,:)'"/1 -> dotprod959/1
  dotprod959/1 -> Mux/959
  "IW{2,1}(960,:)'"/1 -> dotprod960/1
  dotprod960/1 -> Mux/960
  "IW{2,1}(961,:)'"/1 -> dotprod961/1
  dotprod961/1 -> Mux/961
  "IW{2,1}(962,:)'"/1 -> dotprod962/1
  dotprod962/1 -> Mux/962
  "IW{2,1}(963,:)'"/1 -> dotprod963/1
  dotprod963/1 -> Mux/963
  "IW{2,1}(964,:)'"/1 -> dotprod964/1
  dotprod964/1 -> Mux/964
  "IW{2,1}(965,:)'"/1 -> dotprod965/1
  dotprod965/1 -> Mux/965
  "IW{2,1}(966,:)'"/1 -> dotprod966/1
  dotprod966/1 -> Mux/966
  "IW{2,1}(967,:)'"/1 -> dotprod967/1
  dotprod967/1 -> Mux/967
  "IW{2,1}(968,:)'"/1 -> dotprod968/1
  dotprod968/1 -> Mux/968
  "IW{2,1}(969,:)'"/1 -> dotprod969/1
  dotprod969/1 -> Mux/969
  "IW{2,1}(970,:)'"/1 -> dotprod970/1
  dotprod970/1 -> Mux/970
  "IW{2,1}(971,:)'"/1 -> dotprod971/1
  dotprod971/1 -> Mux/971
  "IW{2,1}(972,:)'"/1 -> dotprod972/1
  dotprod972/1 -> Mux/972
  "IW{2,1}(973,:)'"/1 -> dotprod973/1
  dotprod973/1 -> Mux/973
  "IW{2,1}(974,:)'"/1 -> dotprod974/1
  dotprod974/1 -> Mux/974
  "IW{2,1}(975,:)'"/1 -> dotprod975/1
  dotprod975/1 -> Mux/975
  "IW{2,1}(976,:)'"/1 -> dotprod976/1
  dotprod976/1 -> Mux/976
  "IW{2,1}(977,:)'"/1 -> dotprod977/1
  dotprod977/1 -> Mux/977
  "IW{2,1}(978,:)'"/1 -> dotprod978/1
  dotprod978/1 -> Mux/978
  "IW{2,1}(979,:)'"/1 -> dotprod979/1
  dotprod979/1 -> Mux/979
  "IW{2,1}(980,:)'"/1 -> dotprod980/1
  dotprod980/1 -> Mux/980
  "IW{2,1}(981,:)'"/1 -> dotprod981/1
  dotprod981/1 -> Mux/981
  "IW{2,1}(982,:)'"/1 -> dotprod982/1
  dotprod982/1 -> Mux/982
  "IW{2,1}(983,:)'"/1 -> dotprod983/1
  dotprod983/1 -> Mux/983
  "IW{2,1}(984,:)'"/1 -> dotprod984/1
  dotprod984/1 -> Mux/984
  "IW{2,1}(985,:)'"/1 -> dotprod985/1
  dotprod985/1 -> Mux/985
  "IW{2,1}(986,:)'"/1 -> dotprod986/1
  dotprod986/1 -> Mux/986
  "IW{2,1}(987,:)'"/1 -> dotprod987/1
  dotprod987/1 -> Mux/987
  "IW{2,1}(988,:)'"/1 -> dotprod988/1
  dotprod988/1 -> Mux/988
  "IW{2,1}(989,:)'"/1 -> dotprod989/1
  dotprod989/1 -> Mux/989
  "IW{2,1}(990,:)'"/1 -> dotprod990/1
  dotprod990/1 -> Mux/990
  "IW{2,1}(991,:)'"/1 -> dotprod991/1
  dotprod991/1 -> Mux/991
  "IW{2,1}(992,:)'"/1 -> dotprod992/1
  dotprod992/1 -> Mux/992
  "IW{2,1}(993,:)'"/1 -> dotprod993/1
  dotprod993/1 -> Mux/993
  "IW{2,1}(994,:)'"/1 -> dotprod994/1
  dotprod994/1 -> Mux/994
  "IW{2,1}(995,:)'"/1 -> dotprod995/1
  dotprod995/1 -> Mux/995
  "IW{2,1}(996,:)'"/1 -> dotprod996/1
  dotprod996/1 -> Mux/996
  "IW{2,1}(997,:)'"/1 -> dotprod997/1
  dotprod997/1 -> Mux/997
  "IW{2,1}(998,:)'"/1 -> dotprod998/1
  dotprod998/1 -> Mux/998
  "IW{2,1}(999,:)'"/1 -> dotprod999/1
  dotprod999/1 -> Mux/999
  "IW{2,1}(1000,:)'"/1 -> dotprod1000/1
  dotprod1000/1 -> Mux/1000
  "IW{2,1}(1001,:)'"/1 -> dotprod1001/1
  dotprod1001/1 -> Mux/1001
  Mux/1 -> "lz{2,1}"/1
